simulink model "first_quadrant_chopper"  (R2021b)
settings: Solver=ode23tb  StartTime=0.0  StopTime=10.0  MaxStep=1e-4  RelTol=1e-3
libraries: spsDCVoltageSourceLib x1, spsMeanLib x1, spsSeriesRLCBranchLib x1, spsVoltageMeasurementLib x1, spsDiodeLib x1, spspowerguiLib x1, spsIGBTLib x1
settings Model: Creator=mohamednasser  LastModifiedBy=mohamednasser

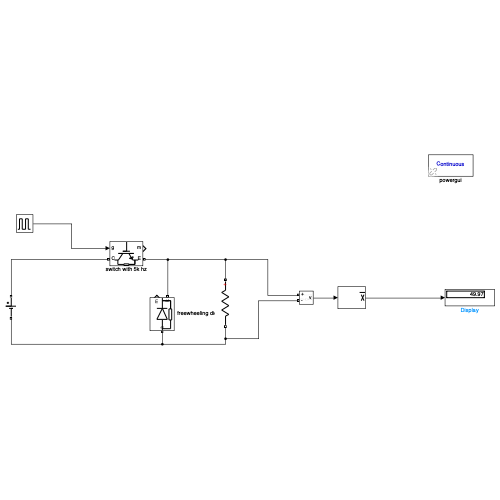
[thumbnail: Simulink's stored preview of the top-level diagram]
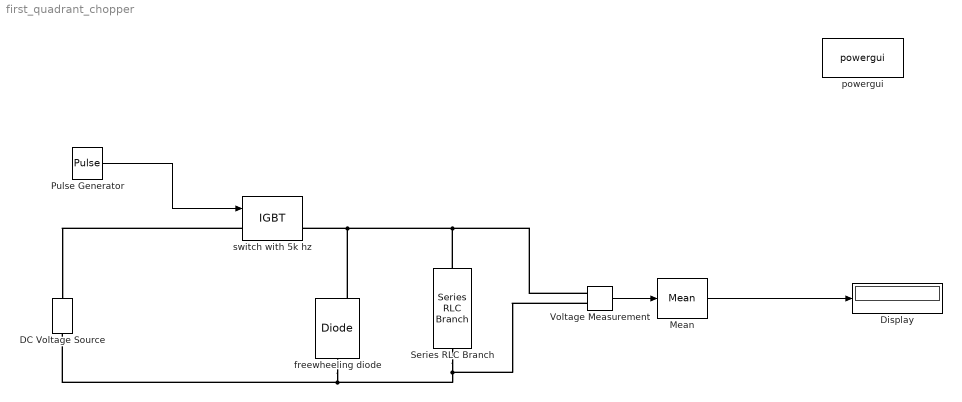
== system first_quadrant_chopper ==
  DC Voltage Source : spsDCVoltageSourceLib/DC Voltage Source  Amplitude=100  Measurements=None
  Display : Display
  Mean : spsMeanLib/Mean  Freq=50  Vinit=0  Ts=0
  Pulse Generator : DiscretePulseGenerator  PulseType=Time based  Period=2e-4  PulseWidth=50
  Series RLC Branch : spsSeriesRLCBranchLib/Series RLC Branch  LConnTagsString=__new0  RConnTagsString=__new0  BranchType=R  Resistance=10  Inductance=1e-3  SetiL0=off  InitialCurrent=0  Capacitance=1e-6  Setx0=off  InitialVoltage=0  Measurements=None
  Voltage Measurement : spsVoltageMeasurementLib/Voltage Measurement  PhasorSimulation=off  OutputType=Complex  PSBequivalent=0
  freewheeling diode : spsDiodeLib/Diode  Ron=0.001  Lon=0  Vf=0.8  IC=0  UseSnubber=0  Rs=500  Cs=250e-9  Measurements=on
  powergui : spspowerguiLib/powergui  Priority=1  SimulationMode=Continuous  SampleTime=50e-6  frequency=60  Iterations=50  frequencyindice=0  Pbase=100e6  ErrMax=1e-4  UnitsV=kV  UnitsW=MW  buscounter=0  FunctionMessages=off  echomessages=off  EnableUseOfTLC=off  CurrentSourceSwitches=off  DisableSnubberDevices=off  DisableRonSwitches=off  DisableVfSwitches=off  DisplayEquations=off  AutomaticDiscreteSolvers=off  SolverType=Tustin/Backward Euler (TBE)  Interpol=off  ExternalGateDelay=off  methode=off  Ts=100  x0status=blocks  SPID=on  SwTol=0  HookPort=off  NonlinearTolerance=1e-4  nMaxIteration=100  ContinueOnMaxIteration=off  RestoreLinks=warning  ResistiveCurrentMeasurement=off  Frange=[0:2:500]  Ylog=off  Xlog=on  ShowGrid=off  save=off  variable=ZData  structure=0  ZoomFFT=off  StartTime=0.0  cycles=1  DisplayStyle=1  fundamental=60  FreqAxis=off  MaxFrequency=1000  frequencyindicesteady=1  RmsSteady=1  display=off
  switch with 5k hz : spsIGBTLib/IGBT  Ron=0.001  Lon=0  Vf=1  Tf=1e-6  Tt=2e-6  IC=0  Rs=1e5  Cs=inf  Measurements=on
  wires:
  Mean/1 -> Display/1
  Pulse Generator/1 -> switch with 5k hz/1
  Voltage Measurement/1 -> Mean/1
  connections:
  switch with 5k hz/LConn1 -- DC Voltage Source/RConn1
  Series RLC Branch/RConn1 -- freewheeling diode/LConn1 -- DC Voltage Source/LConn1 -- Voltage Measurement/LConn2
  Series RLC Branch/LConn1 -- freewheeling diode/RConn1 -- switch with 5k hz/RConn1 -- Voltage Measurement/LConn1
